simulink model "dynamicabsorber1"  (R2021a)
settings: Solver=VariableStepAuto  StartTime=0.0  StopTime=10.0  RelTol=1e-3
undefined symbols (not defined in the file): k
settings Model: Creator=Nida  LastModifiedBy=Nida

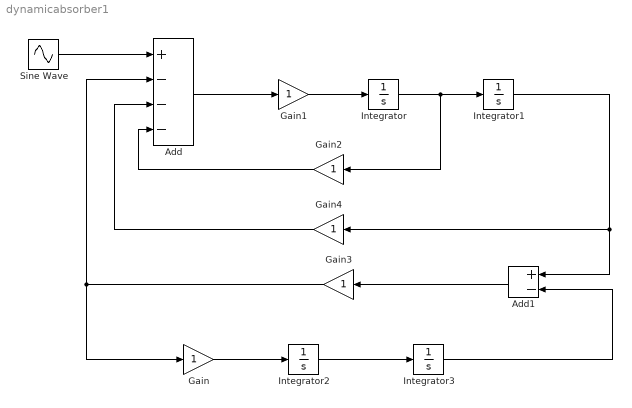
== system dynamicabsorber1 ==
  Add : Sum  Inputs=+---
  Add1 : Sum  Inputs=+-
  Gain{,2..4} (4 alike) : Gain
  Gain1 : Gain  OutMax=k
  Integrator{,1..3} (4 alike) : Integrator
  Sine Wave : Sin  SampleTime=0
  wires:
  Add/1 -> Gain1/1
  Integrator/1 -> Gain2/1, Integrator1/1
  Gain2/1 -> Add/4
  Gain4/1 -> Add/3
  Gain3/1 -> Gain/1, Add/2
  Integrator1/1 -> Add1/1, Gain4/1
  Add1/1 -> Gain3/1
  Gain/1 -> Integrator2/1
  Integrator2/1 -> Integrator3/1
  Integrator3/1 -> Add1/2
  Sine Wave/1 -> Add/1
  Gain1/1 -> Integrator/1
